simulink model "ITPW26_SHE"  (R2015b)
settings: Solver=VariableStepAuto  SolverMode=SingleTasking  StartTime=0.0  StopTime=1  RelTol=1e-3
libraries: powerlib x21, simulink x8, powerlib_meascontrol x4
settings Model: Creator=SPIRO-POWER  LastModifiedBy=SPIRO-POWER
settings DataIOCC: LimitDataPoints=off
settings DebuggingCC: AllowSymbolicDim=on  SFUnexpectedBacktrackingDiag=error  SFNoUnconditionalDefaultTransitionDiag=error
settings ModelReferenceCC: PropagateSignalLabelsOutOfModel=on
settings GRTTargetCC: TargetLangStandard=C99 (ISO)
settings ConfigComp: CovMetricSettings=dwe  CovHtmlReporting=off  CovSaveCumulativeToWorkspaceVar=off  CovSaveSingleToWorkspaceVar=off  CovModelRefEnable=Off  CovExternalEMLEnable=on

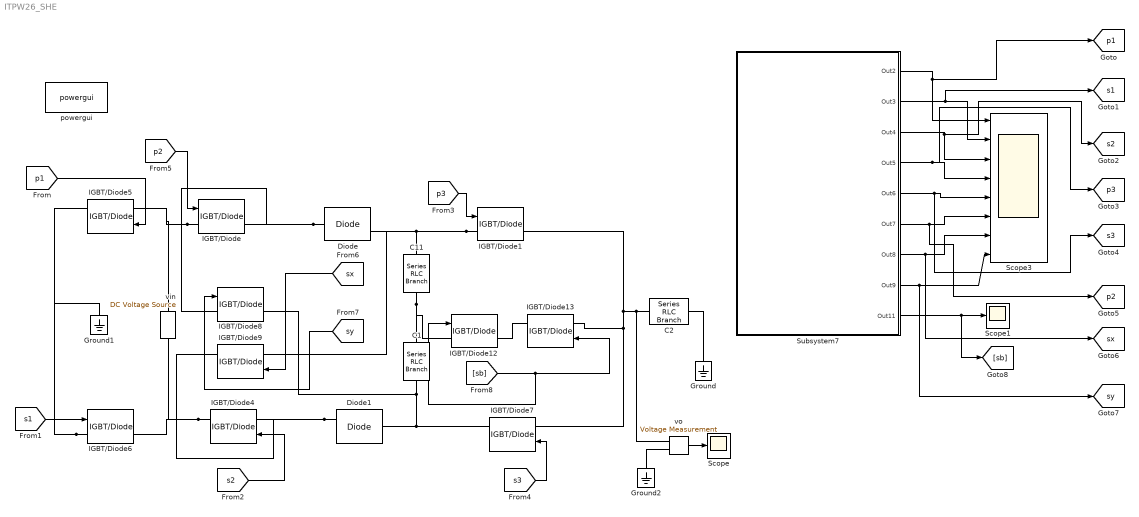
== system ITPW26_SHE ==
  C1 : powerlib/Elements/Series RLC Branch  LConnTagsString=__new0  RConnTagsString=__new0  BranchType=C  Resistance=1  Inductance=1e-3  SetiL0=off  InitialCurrent=0  Capacitance=10000e-6  Setx0=off  InitialVoltage=0  Measurements=None
  C11 : powerlib/Elements/Series RLC Branch  LConnTagsString=__new0  RConnTagsString=__new0  BranchType=C  Resistance=1  Inductance=1e-3  SetiL0=off  InitialCurrent=0  Capacitance=10000e-6  Setx0=off  InitialVoltage=0  Measurements=None
  C2 : powerlib/Elements/Series RLC Branch  LConnTagsString=__new0  RConnTagsString=__new0  BranchType=R  Resistance=250  Inductance=0.01  SetiL0=off  InitialCurrent=0  Capacitance=100e-6  Setx0=off  InitialVoltage=0  Measurements=None
  Diode : powerlib/Power Electronics/Diode  Ron=0.001  Lon=0  Vf=0.8  IC=0  UseSnubber=off  Rs=500  Cs=250e-9  Measurements=on
  Diode1 : powerlib/Power Electronics/Diode  Ron=0.001  Lon=0  Vf=0.8  IC=0  UseSnubber=off  Rs=500  Cs=250e-9  Measurements=on
  Ground : powerlib/Elements/Ground  LConnTagsString=a
  Ground1 : powerlib/Elements/Ground  LConnTagsString=a
  Ground2 : powerlib/Elements/Ground  LConnTagsString=a
  IGBT/Diode{,1,4..9,12..13} (10 alike) : powerlib/Power Electronics/IGBT//Diode  Ron=1e-3  Rs=1e5  Cs=inf  Measurements=on
  Scope : Scope
  Scope1 : Scope
  Scope3 : Scope  NumInputPorts=8
  Subsystem7 : Subsystem
  powergui : powerlib/powergui  Priority=1  SimulationMode=Continuous  SolverType=Tustin/Backward Euler (TBE)  SampleTime=50e-6  frequency=60  SPID=off  DisableSnubberDevices=off  DisableRonSwitches=off  DisableVfSwitches=off  SwTol=0  DisplayEquations=off  Interpol=off  ExternalGateDelay=off  methode=off  Ts=100  FunctionMessages=off  echomessages=off  HookPort=off  EnableUseOfTLC=off  x0status=blocks  frequencyindice=0  Pbase=100e6  ErrMax=1e-4  Iterations=50  UnitsV=kV  UnitsW=MW  buscounter=0  RestoreLinks=warning  ResistiveCurrentMeasurement=off  Frange=[0:2:500]  Ylog=off  Xlog=on  ShowGrid=off  save=off  variable=ZData  structure=v2  ZoomFFT=on  StartTime=0.5  cycles=5  DisplayStyle=1  fundamental=50  FreqAxis=off  MaxFrequency=1000  frequencyindicesteady=1  RmsSteady=1  display=off
  vin : powerlib/Electrical Sources/DC Voltage Source  Amplitude=100  Measurements=None
  vo : powerlib/Measurements/Voltage Measurement  PhasorSimulation=off  OutputType=Complex  PSBequivalent=0
  tag scope: p1=global, p2=global, p3=global, s1=global, s2=global, s3=global, sx=global, sy=global
  wires:
  [sx] -> IGBT/Diode9/1
  [s3] -> IGBT/Diode7/1
  Subsystem7/2(Out3) -> [s1], Scope3/2
  Subsystem7/9(Out11) -> [sb], Scope1/1
  [p3] -> IGBT/Diode1/1
  Subsystem7/5(Out6) -> [s3], Scope3/5
  [s1] -> IGBT/Diode6/1
  [sb] -> IGBT/Diode12/1, IGBT/Diode13/1
  Subsystem7/7(Out8) -> [sx], Scope3/7
  [sy] -> IGBT/Diode8/1
  Subsystem7/4(Out5) -> [p3], Scope3/4
  vo/1 -> Scope/1
  Subsystem7/3(Out4) -> [s2], Scope3/3
  [s2] -> IGBT/Diode4/1
  Subsystem7/6(Out7) -> [p2], Scope3/6
  [p1] -> IGBT/Diode5/1
  [p2] -> IGBT/Diode/1
  Subsystem7/1(Out2) -> [p1], Scope3/1
  Subsystem7/8(Out9) -> [sy], Scope3/8
  connections:
  IGBT/Diode1/LConn1 -- C11/LConn1 -- Diode/RConn1 -- IGBT/Diode9/LConn1
  C2/LConn1 -- vo/LConn1 -- IGBT/Diode1/RConn1 -- IGBT/Diode13/LConn1 -- IGBT/Diode7/LConn1
  C1/RConn1 -- Diode1/LConn1 -- IGBT/Diode7/RConn1 -- IGBT/Diode8/RConn1
  IGBT/Diode6/LConn1 -- IGBT/Diode5/RConn1 -- Ground1/LConn1
  Diode/LConn1 -- IGBT/Diode/RConn1 -- IGBT/Diode8/LConn1
  C11/RConn1 -- C1/LConn1 -- IGBT/Diode12/LConn1
  IGBT/Diode4/RConn1 -- IGBT/Diode6/RConn1 -- vin/LConn1
  Diode1/RConn1 -- IGBT/Diode4/LConn1 -- IGBT/Diode9/RConn1
  IGBT/Diode/LConn1 -- IGBT/Diode5/LConn1 -- vin/RConn1
  Ground/LConn1 -- C2/RConn1
  IGBT/Diode13/RConn1 -- IGBT/Diode12/RConn1
  Ground2/LConn1 -- vo/LConn2

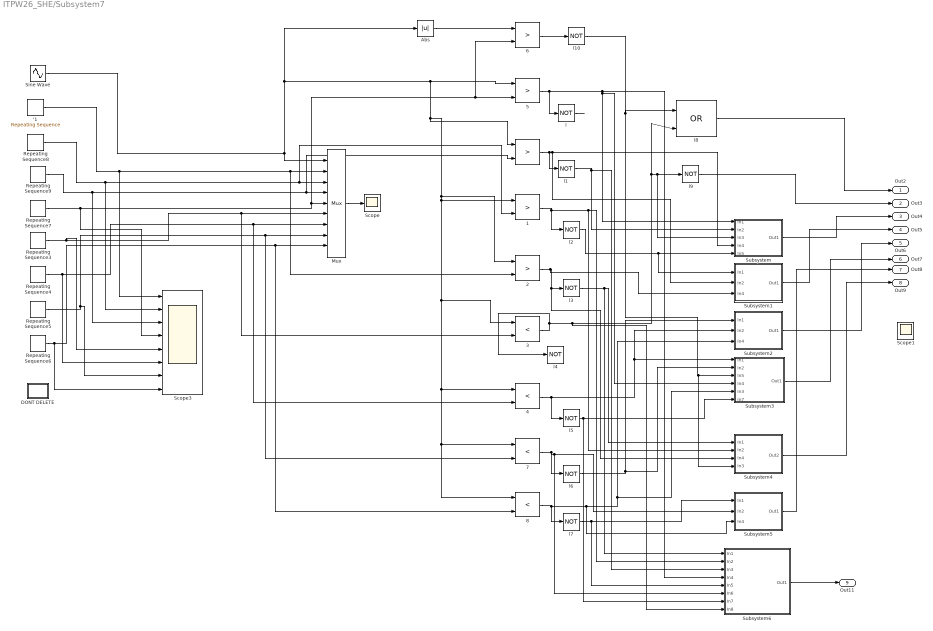
== system ITPW26_SHE/Subsystem7 ==
   {,1..2,5..6} (5 alike) : RelationalOperator  Operator=>  OutDataTypeStr=boolean
   {3..4,7..8} (4 alike) : RelationalOperator  Operator=<  OutDataTypeStr=boolean
  '1 : simulink/Sources/Repeating Sequence  rep_seq_t=[0 0.001/2 0.001]  rep_seq_y=[3 4 3]
  Abs : Abs
  DONT DELETE : Subsystem
  Mux : Mux  Inputs=9
  Repeating Sequence3 : simulink/Sources/Repeating Sequence  rep_seq_t=[0 0.001/2 0.001]  rep_seq_y=[0 -1 0]
  Repeating Sequence4 : simulink/Sources/Repeating Sequence  rep_seq_t=[0 0.001/2 0.001]  rep_seq_y=[-1 -2 -1]
  Repeating Sequence5 : simulink/Sources/Repeating Sequence  rep_seq_t=[0 0.001/2 0.001]  rep_seq_y=[-2 -3 -2]
  Repeating Sequence6 : simulink/Sources/Repeating Sequence  rep_seq_t=[0 0.001/2 0.001]  rep_seq_y=[-3 -4 -3]
  Repeating Sequence7 : simulink/Sources/Repeating Sequence  rep_seq_t=[0 0.001/2 0.001]  rep_seq_y=[0 1 0]
  Repeating Sequence8 : simulink/Sources/Repeating Sequence  rep_seq_t=[0 0.001/2 0.001]  rep_seq_y=[2 3 2]
  Repeating Sequence9 : simulink/Sources/Repeating Sequence  rep_seq_t=[0 0.001/2 0.001]  rep_seq_y=[1 2 1]
  Scope : Scope
  Scope1 : Scope
  Scope3 : Scope  NumInputPorts=8
  Sine Wave : Sin  Amplitude=4  Frequency=2*pi*50  SampleTime=0
  Subsystem : Subsystem
  Subsystem1 : Subsystem
  Subsystem2 : Subsystem
  Subsystem3 : Subsystem
  Subsystem4 : Subsystem
  Subsystem5 : Subsystem
  Subsystem6 : Subsystem
  l{,1..7,9..10} (10 alike) : Logic  Operator=NOT  IconShape=distinctive  AllPortsSameDT=off  OutDataTypeStr=boolean
  l8 : Logic  Operator=OR  IconShape=distinctive  AllPortsSameDT=off  OutDataTypeStr=boolean
  Out2 : Outport
  Out3 : Outport  Port=2
  Out4 : Outport  Port=3
  Out5 : Outport  Port=4
  Out6 : Outport  Port=5
  Out7 : Outport  Port=6
  Out8 : Outport  Port=7
  Out9 : Outport  Port=8
  Out11 : Outport  Port=9
  wires:
  Repeating Sequence7/1 -> Scope3/4, " 6"/2, " 5"/2, Mux/5
  " 8"/1 -> Subsystem5/3(In4), Subsystem3/5(In3), Subsystem2/3(In4), l7/1
  " 3"/1 -> Subsystem6/8(In8), Subsystem/3(In3), l9/1, l8/2, l4/1
  Subsystem3/1(Out1) -> Out7/1
  " 4"/1 -> Subsystem2/2(In2), Subsystem3/1(In1), l5/1
  l7/1 -> Subsystem6/5(In5), Subsystem5/1(In1)
  Mux/1 -> Scope/1
  " 7"/1 -> Subsystem5/2(In2), Subsystem6/6(In6), l6/1
  '1/1 -> Scope3/1, " 2"/2, Mux/2
  l5/1 -> Subsystem6/7(In7), Subsystem3/6(In7)
  Subsystem/1(Out1) -> Out4/1
  l3/1 -> Subsystem6/1(In1), Subsystem4/1(In1)
  " 1"/1 -> Subsystem6/2(In2), Subsystem4/2(In2), l2/1
  l1/1 -> Subsystem6/3(In3), Subsystem/2(In2)
  " 5"/1 -> Subsystem6/4(In4), Subsystem3/4(In4), Subsystem/1(In1), l/1
  Subsystem1/1(Out1) -> Out5/1
  l/1 -> ?
  Repeating Sequence9/1 -> Scope3/3, " "/2, Mux/4
  Sine Wave/1 -> Mux/1, " 2"/1, " 3"/1, " 8"/1, " 7"/1, " 4"/1, " 1"/1, " "/1, " 5"/1, Abs/1
  " 6"/1 -> l10/1
  " 2"/1 -> Subsystem1/3(In4), Subsystem4/3(In4), l3/1
  l2/1 -> Subsystem1/1(In1), Subsystem/5(In5)
  Abs/1 -> " 6"/1
  l6/1 -> Subsystem3/2(In2), Subsystem2/1(In1)
  Subsystem6/1(Out1) -> Out11/1
  Repeating Sequence8/1 -> Scope3/2, " 1"/2, Mux/3
  Subsystem2/1(Out1) -> Out6/1
  l9/1 -> Out3/1
  l8/1 -> Out2/1
  " "/1 -> Subsystem1/2(In2), Subsystem/4(In4), l1/1
  Repeating Sequence3/1 -> Scope3/5, " 3"/2, Mux/6
  Repeating Sequence4/1 -> Scope3/6, " 4"/2, Mux/7
  Repeating Sequence5/1 -> Scope3/7, " 7"/2, Mux/8
  Repeating Sequence6/1 -> Scope3/8, " 8"/2, Mux/9
  l10/1 -> Subsystem4/4(In3), Subsystem3/3(In5), l8/1
  Subsystem4/1(Out2) -> Out9/1
  Subsystem5/1(Out1) -> Out8/1

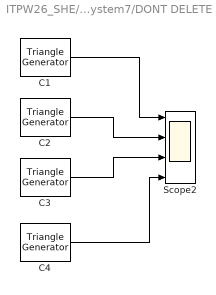
== system ITPW26_SHE/Subsystem7/DONT DELETE ==
  C1 : powerlib_meascontrol/Pulse & Signal Generators/Triangle Generator  Freq=1e3  Phase=180  Ts=0
  C2 : powerlib_meascontrol/Pulse & Signal Generators/Triangle Generator  Freq=1e3  Phase=90  Ts=0
  C3 : powerlib_meascontrol/Pulse & Signal Generators/Triangle Generator  Freq=1e3  Phase=90  Ts=0
  C4 : powerlib_meascontrol/Pulse & Signal Generators/Triangle Generator  Freq=1e3  Phase=90  Ts=0
  Scope2 : Scope  NumInputPorts=4
  wires:
  C3/1 -> Scope2/3
  C1/1 -> Scope2/1
  C4/1 -> Scope2/4
  C2/1 -> Scope2/2

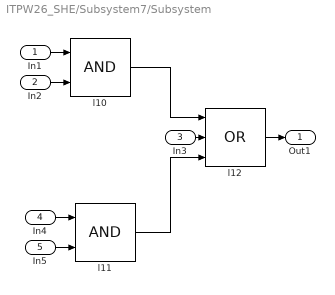
== system ITPW26_SHE/Subsystem7/Subsystem ==
  In1 : Inport
  In2 : Inport  Port=2
  In3 : Inport  Port=3
  In4 : Inport  Port=4
  In5 : Inport  Port=5
  l10 : Logic  IconShape=distinctive  AllPortsSameDT=off  OutDataTypeStr=boolean
  l11 : Logic  IconShape=distinctive  AllPortsSameDT=off  OutDataTypeStr=boolean
  l12 : Logic  Operator=OR  Inputs=3  IconShape=distinctive  AllPortsSameDT=off  OutDataTypeStr=boolean
  Out1 : Outport
  wires:
  In3/1 -> l12/2
  l11/1 -> l12/3
  In4/1 -> l11/1
  l12/1 -> Out1/1
  In5/1 -> l11/2
  In1/1 -> l10/1
  In2/1 -> l10/2
  l10/1 -> l12/1

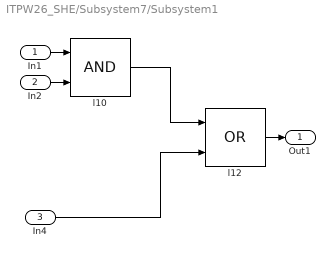
== system ITPW26_SHE/Subsystem7/Subsystem1 ==
  In1 : Inport
  In2 : Inport  Port=2
  In4 : Inport  Port=3
  l10 : Logic  IconShape=distinctive  AllPortsSameDT=off  OutDataTypeStr=boolean
  l12 : Logic  Operator=OR  IconShape=distinctive  AllPortsSameDT=off  OutDataTypeStr=boolean
  Out1 : Outport
  wires:
  l10/1 -> l12/1
  In2/1 -> l10/2
  In1/1 -> l10/1
  l12/1 -> Out1/1
  In4/1 -> l12/2

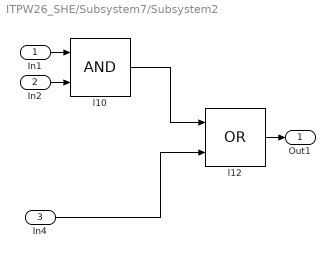
== system ITPW26_SHE/Subsystem7/Subsystem2 ==
  In1 : Inport
  In2 : Inport  Port=2
  In4 : Inport  Port=3
  l10 : Logic  IconShape=distinctive  AllPortsSameDT=off  OutDataTypeStr=boolean
  l12 : Logic  Operator=OR  IconShape=distinctive  AllPortsSameDT=off  OutDataTypeStr=boolean
  Out1 : Outport
  wires:
  In4/1 -> l12/2
  l12/1 -> Out1/1
  In1/1 -> l10/1
  In2/1 -> l10/2
  l10/1 -> l12/1

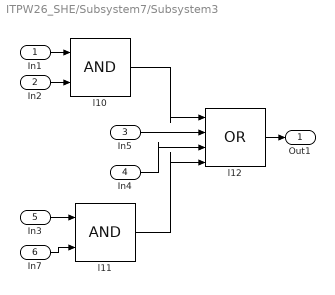
== system ITPW26_SHE/Subsystem7/Subsystem3 ==
  In1 : Inport
  In2 : Inport  Port=2
  In5 : Inport  Port=3
  In4 : Inport  Port=4
  In3 : Inport  Port=5
  In7 : Inport  Port=6
  l10 : Logic  IconShape=distinctive  AllPortsSameDT=off  OutDataTypeStr=boolean
  l11 : Logic  IconShape=distinctive  AllPortsSameDT=off  OutDataTypeStr=boolean
  l12 : Logic  Operator=OR  Inputs=4  IconShape=distinctive  AllPortsSameDT=off  OutDataTypeStr=boolean
  Out1 : Outport
  wires:
  l10/1 -> l12/1
  In2/1 -> l10/2
  In1/1 -> l10/1
  l12/1 -> Out1/1
  In3/1 -> l11/1
  In5/1 -> l12/2
  l11/1 -> l12/4
  In4/1 -> l12/3
  In7/1 -> l11/2

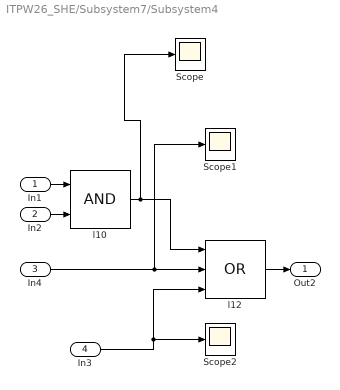
== system ITPW26_SHE/Subsystem7/Subsystem4 ==
  In1 : Inport
  In2 : Inport  Port=2
  In4 : Inport  Port=3
  In3 : Inport  Port=4
  Scope : Scope
  Scope1 : Scope
  Scope2 : Scope
  l10 : Logic  IconShape=distinctive  AllPortsSameDT=off  OutDataTypeStr=boolean
  l12 : Logic  Operator=OR  Inputs=3  IconShape=distinctive  AllPortsSameDT=off  OutDataTypeStr=boolean
  Out2 : Outport
  wires:
  l10/1 -> Scope/1, l12/1
  In2/1 -> l10/2
  In1/1 -> l10/1
  l12/1 -> Out2/1
  In4/1 -> Scope1/1, l12/2
  In3/1 -> Scope2/1, l12/3

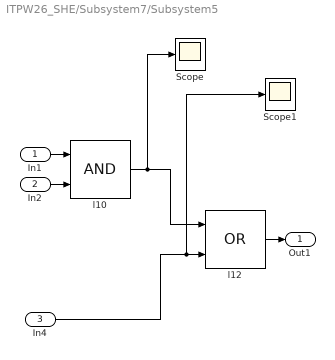
== system ITPW26_SHE/Subsystem7/Subsystem5 ==
  In1 : Inport
  In2 : Inport  Port=2
  In4 : Inport  Port=3
  Scope : Scope
  Scope1 : Scope
  l10 : Logic  IconShape=distinctive  AllPortsSameDT=off  OutDataTypeStr=boolean
  l12 : Logic  Operator=OR  IconShape=distinctive  AllPortsSameDT=off  OutDataTypeStr=boolean
  Out1 : Outport
  wires:
  l10/1 -> Scope/1, l12/1
  In2/1 -> l10/2
  In1/1 -> l10/1
  l12/1 -> Out1/1
  In4/1 -> Scope1/1, l12/2

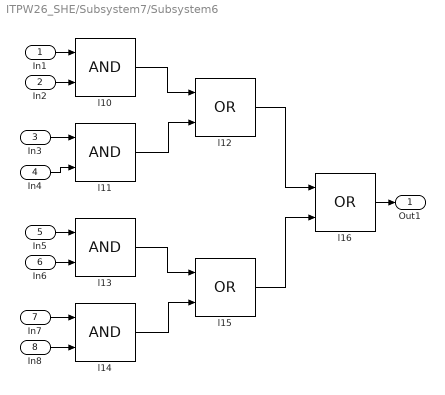
== system ITPW26_SHE/Subsystem7/Subsystem6 ==
  In1 : Inport
  In2 : Inport  Port=2
  In3 : Inport  Port=3
  In4 : Inport  Port=4
  In5 : Inport  Port=5
  In6 : Inport  Port=6
  In7 : Inport  Port=7
  In8 : Inport  Port=8
  l{10..11,13..14} (4 alike) : Logic  IconShape=distinctive  AllPortsSameDT=off  OutDataTypeStr=boolean
  l12 : Logic  Operator=OR  IconShape=distinctive  AllPortsSameDT=off  OutDataTypeStr=boolean
  l15 : Logic  Operator=OR  IconShape=distinctive  AllPortsSameDT=off  OutDataTypeStr=boolean
  l16 : Logic  Operator=OR  IconShape=distinctive  AllPortsSameDT=off  OutDataTypeStr=boolean
  Out1 : Outport
  wires:
  l14/1 -> l15/2
  In8/1 -> l14/2
  l13/1 -> l15/1
  l15/1 -> l16/2
  In2/1 -> l10/2
  l12/1 -> l16/1
  l16/1 -> Out1/1
  In6/1 -> l13/2
  In7/1 -> l14/1
  l11/1 -> l12/2
  l10/1 -> l12/1
  In5/1 -> l13/1
  In1/1 -> l10/1
  In4/1 -> l11/2
  In3/1 -> l11/1
